simulink model "beta_estimator_velocity_driftingcar"  (R2017a)
settings: Solver=FixedStepAuto  StartTime=0.0  StopTime=10.0  FixedStep=0.01  RelTol=1e-3
undefined symbols (not defined in the file or in its folder): DiscIntNeverNeededParam
libraries: robotlib x4
settings Model: Creator=bascetta  LastModifiedBy=marco
settings OptimizationCC: PassReuseOutputArgsAs=Individual arguments  MaxStackSize=64
settings DebuggingCC: ParameterTunabilityLossMsg=error
settings HardwareCC: ProdBitPerPointer=32  ProdBitPerSizeT=32  ProdBitPerPtrDiffT=32  ProdLargestAtomicFloat=None  ProdIntDivRoundTo=Undefined  ProdEndianess=Unspecified  ProdWordSize=32  ProdHWDeviceType=Generic->Unspecified (assume 32-bit Generic)
settings SFSimCC: MATLABDynamicMemAlloc=off
settings RTWCC: SystemTargetFile=ert.tlc  HardwareBoard=Robot Operating System (ROS)  TLCOptions="-aInlineSetEventsForThisBaseRateFcn=TLC_FALSE -aSuppressMultiTaskScheduler=TLC_FALSE  -aRateBasedStepFcn=0"  TemplateMakefile=ert_default_tmf  Description=Embedded Coder  GenerateReport=on  Toolchain=Catkin  IncludeHyperlinkInReport=on  LaunchReport=on  TargetLang=C++  GenerateTraceInfo=on  GenerateTraceReport=on  GenerateTraceReportSl=on  GenerateTraceReportSf=on  GenerateTraceReportEml=on
settings CodeAppCC: ForceParamTrailComments=on  IgnoreCustomStorageClasses=off  OperatorAnnotations=on  SimulinkDataObjDesc=on  SFDataObjDesc=on  MATLABFcnDesc=on  InsertBlockDesc=on  MATLABSourceComments=on
settings ConfigComp: CovScope=ReferencedModels  CovIncludeTopModel=off

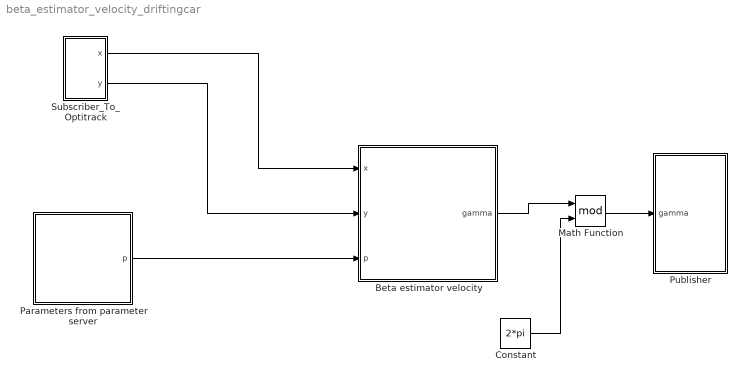
== system beta_estimator_velocity_driftingcar ==
  Beta estimator velocity : Subsystem
  Constant : Constant  Value=2*pi
  Math Function : Math  Operator=mod  OutputSignalType=real  SaturateOnIntegerOverflow=on
  Parameters from parameter server : Subsystem
  Publisher : Subsystem
  Subscriber_To_Optitrack : Subsystem
  wires:
  Parameters from parameter server/1(p) -> Beta estimator velocity/3(p)
  Beta estimator velocity/1(gamma) -> Math Function/1
  Subscriber_To_Optitrack/1(x) -> Beta estimator velocity/1(x)
  Subscriber_To_Optitrack/2(y) -> Beta estimator velocity/2(y)
  Math Function/1 -> Publisher/1(gamma)
  Constant/1 -> Math Function/2

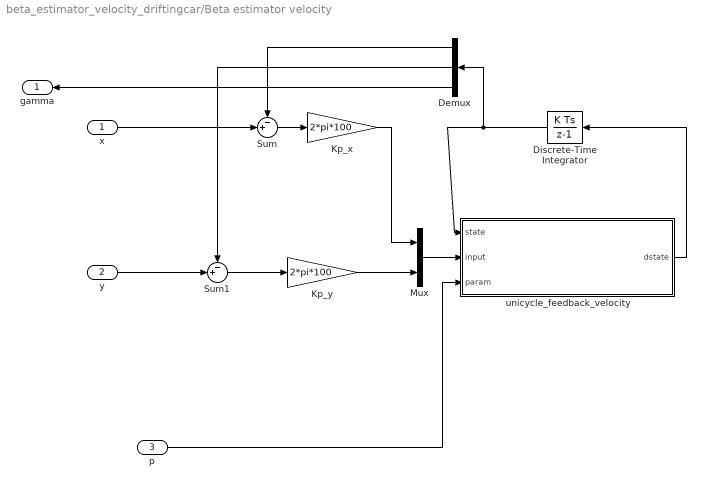
== system beta_estimator_velocity_driftingcar/Beta estimator velocity ==
  x : Inport
  y : Inport  Port=2
  p : Inport  Port=3
  Demux : Demux  Outputs=3
  Discrete-Time Integrator : DiscreteIntegrator  InitialConditionSetting=State (most efficient)  SampleTime=-1  ICPrevOutput=DiscIntNeverNeededParam  ICPrevScaledInput=DiscIntNeverNeededParam
  Kp_x : Gain  Gain=2*pi*100
  Kp_y : Gain  Gain=2*pi*100
  Mux : Mux  Inputs=2
  Sum : Sum  Inputs=-+|
  Sum1 : Sum  Inputs=-+|
  unicycle_feedback_velocity : MATLAB Function  TreatAsAtomicUnit=on
  gamma : Outport
  wires:
  Demux/3 -> gamma/1
  y/1 -> Sum1/2
  Demux/1 -> Sum/1
  Sum1/1 -> Kp_y/1
  Kp_y/1 -> Mux/2
  Kp_x/1 -> Mux/1
  Mux/1 -> unicycle_feedback_velocity/2(input)
  p/1 -> unicycle_feedback_velocity/3(param)
  Sum/1 -> Kp_x/1
  Demux/2 -> Sum1/1
  x/1 -> Sum/2
  unicycle_feedback_velocity/1(dstate) -> Discrete-Time Integrator/1
  Discrete-Time Integrator/1 -> Demux/1, unicycle_feedback_velocity/1(state)

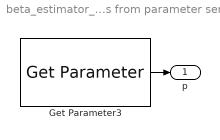
== system beta_estimator_velocity_driftingcar/Parameters from parameter server ==
  Get Parameter3 : robotlib/Get Parameter  SourceLibraryInfo=This block requires Robotics System Toolbox  ParameterSource=Specify your own  ParameterName=/beta_estimator_velocity_driftingcar/p  ParameterType=double  ParameterMaxArrayLength=16  ParameterInitialValue=0.0  SampleTime=-1  ShowErrorCodeOutput=off  ModelName=beta_estimator_velocity_driftingcar  BlockId=ParamGet_beta_estimator_velocity_driftingcar_63
      settings: SourceProductName=Robotics System Toolbox  SourceProductBaseCode=RO
  p : Outport
  wires:
  Get Parameter3/1 -> p/1

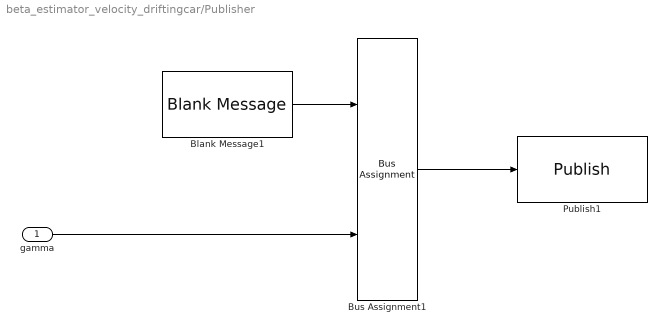
== system beta_estimator_velocity_driftingcar/Publisher ==
  gamma : Inport
  Blank Message1 : robotlib/Blank Message  SourceLibraryInfo=This block requires Robotics System Toolbox  messageType=std_msgs/Float64  SampleTime=inf
      settings: SourceProductBaseCode=RO
  Bus Assignment1 : BusAssignment  AssignedSignals=Data
  Publish1 : robotlib/Publish  SourceLibraryInfo=This block requires Robotics System Toolbox  topicSource=Specify your own  topic=/gamma_estimator_velocity  messageType=std_msgs/Float64  messageQueueLength=1
      settings: SourceProductBaseCode=RO
  wires:
  gamma/1 -> Bus Assignment1/2
  Blank Message1/1 -> Bus Assignment1/1
  Bus Assignment1/1 -> Publish1/1

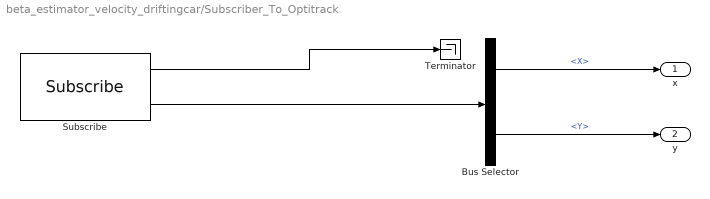
== system beta_estimator_velocity_driftingcar/Subscriber_To_Optitrack ==
  Bus Selector : BusSelector  OutputSignals=Pose.Position.X,Pose.Position.Y
  Subscribe : robotlib/Subscribe  SourceLibraryInfo=This block requires Robotics System Toolbox  topicSource=Specify your own  topic=/car/pose  messageType=geometry_msgs/PoseStamped  sampleTime=-1  messageQueueLength=1
      settings: SourceProductBaseCode=RO
  Terminator : Terminator
  x : Outport
  y : Outport  Port=2
  wires:
  Subscribe/2 -> Bus Selector/1
  Subscribe/1 -> Terminator/1
  Bus Selector/1 -> x/1  "<X>"
  Bus Selector/2 -> y/1  "<Y>"

== matlab function beta_estimator_velocity_driftingcar/Beta estimator velocity/unicycle_feedback_velocity ==
  data: state input size=3; dstate output size=3; input input size=2; param input size=1
function dstate = unicycle_feedback_velocity(state,input,param)

% State and input variables
x     = state(1);
y     = state(2);
gamma = state(3); % theta+beta

vxp   = input(1);
vyp   = input(2);

% Parameters
p = param(1);

% Model equations
dstate = zeros(3,1);
dstate(1) = vxp*cos(gamma)^2+vyp*sin(gamma)*cos(gamma);
dstate(2) = vxp*sin(gamma)*cos(gamma)+vyp*sin(gamma)^2;
dstate(3) = (vyp*cos(gamma)-vxp*sin(gamma))/p;
